simulink model "two_time_domains"  (R2025b)
settings: Solver=ode23tb  StartTime=0.0  StopTime=simlength  MaxStep=tc
undefined symbols (not defined in the file): dead_time_AFE, enable_pwm_phase_corrections, fPWM_AFE, fPWM_INV, ki_align, kp_align, lim_down_align, lim_up_align, omega_base, tc, time_gain_afe_module_1, time_gain_afe_module_2, time_gain_inv_module_1, time_gain_inv_module_2, trgo_th_generator, ts_afe, ts_inv
settings Model: Creator=dbagn  LastModifiedBy=dbagn
settings SolverCC: NumberNewtonIterations=3.0  ZeroCrossControl=DisableAll  AlgebraicLoopSolver=TrustRegion  SolverResetMethod=Robust  AutoInsertRateTranBlk=on
settings DataIOCC: SaveOutput=off  SignalLogging=off  DSMLogging=off  SaveTime=off  ReturnWorkspaceOutputs=off
settings OptimizationCC: ReuseModelBlockBuffer=off
settings DebuggingCC: UnconnectedInputMsg=warning  UnconnectedOutputMsg=warning  UnconnectedLineMsg=warning
settings ModelReferenceCC: UpdateModelReferenceTargets=Force  EnableRefExpFcnMdlSchedulingChecks=on  ParallelModelReferenceMATLABWorkerInit=Copy Base Workspace
settings SFSimCC: CustomCodeUndefinedFunction=ThrowError  DefaultCustomCodeDeterministicFunctions=All
settings RTWCC: GPUComputeCapability=3.5  DLArmComputeVersion=19.05

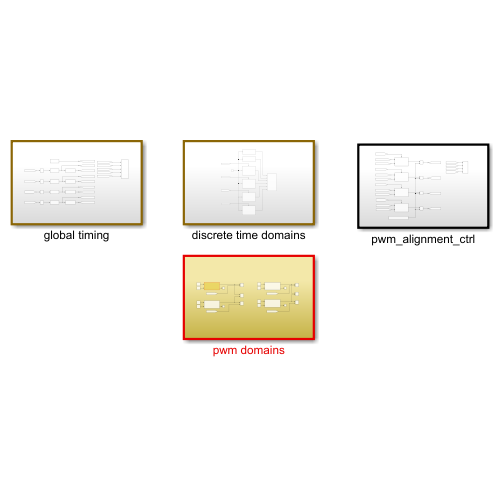
[thumbnail: Simulink's stored preview of the top-level diagram]
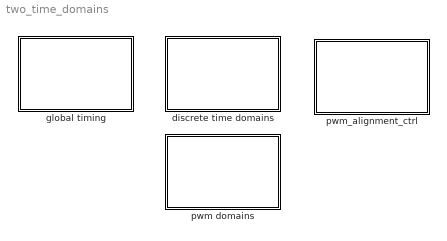
== system two_time_domains ==
  discrete time domains : Subsystem
  global timing : Subsystem
  pwm domains : Subsystem
  pwm_alignment_ctrl : Subsystem

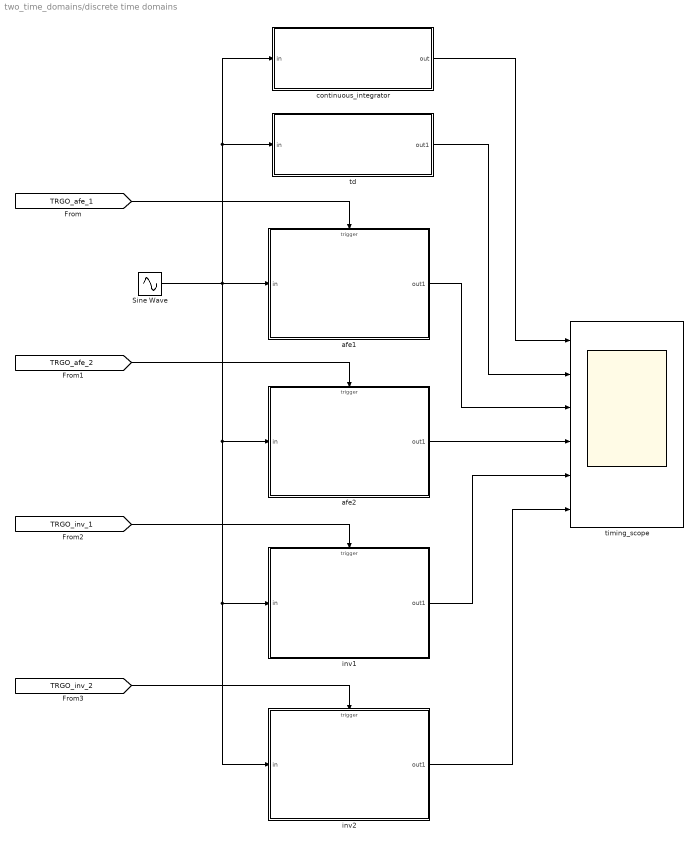
== system two_time_domains/discrete time domains ==
  Sine Wave : Sin  Frequency=omega_base  SampleTime=0
  afe1 : Subsystem
  afe2 : Subsystem
  continuous_integrator : Subsystem
  inv1 : Subsystem
  inv2 : Subsystem
  td : Subsystem
  timing_scope : Scope  NumInputPorts=6
      settings: SampleTime=tc  ActiveDisplayYMinimum=-1.2455953752901299  ActiveDisplayYMaximum=1.2309135739886372
  wires:
  [TRGO_afe_1] -> afe1/Trigger
  [TRGO_afe_2] -> afe2/Trigger
  Sine Wave/1 -> td/1(in), continuous_integrator/1(in), afe1/1(in), inv2/1(in), inv1/1(in), afe2/1(in)
  [TRGO_inv_2] -> inv2/Trigger
  [TRGO_inv_1] -> inv1/Trigger
  afe1/1(out1) -> timing_scope/3
  afe2/1(out1) -> timing_scope/4
  inv1/1(out1) -> timing_scope/5
  inv2/1(out1) -> timing_scope/6
  td/1(out1) -> timing_scope/2
  continuous_integrator/1(out) -> timing_scope/1

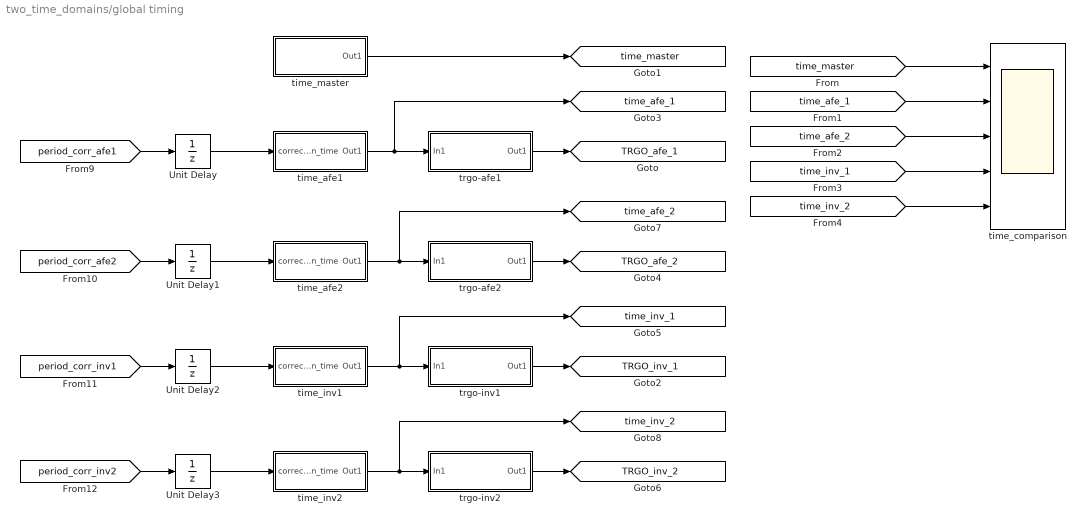
== system two_time_domains/global timing ==
  Unit Delay{,1..3} (4 alike) : UnitDelay  SampleTime=tc  HasFrameUpgradeWarning=on
  time_afe1 : Subsystem  mask{k=time_gain_afe_module_1}
      mask prompts: k "Time Gain"
      mask Display:
      | disp('time-gen');
      | port_label('input', 1, 'crt');
      | port_label('output', 1, 'tout');
  time_afe2 : Subsystem  mask{k=time_gain_afe_module_2}
      mask prompts: k "Time Gain"
      mask Display:
      | disp('time-gen');
      | port_label('input', 1, 'crt');
      | port_label('output', 1, 'tout');
  time_comparison : Scope  NumInputPorts=5
      settings: ActiveDisplayYMinimum=-0.0261093772199036  ActiveDisplayYMaximum=0.23498439497913245  DataLoggingVariableName=ScopeData6
  time_inv1 : Subsystem  mask{k=time_gain_inv_module_1}
      mask prompts: k "Time Gain"
      mask Display:
      | disp('time-gen');
      | port_label('input', 1, 'crt');
      | port_label('output', 1, 'tout');
  time_inv2 : Subsystem  mask{k=time_gain_inv_module_2}
      mask prompts: k "Time Gain"
      mask Display:
      | disp('time-gen');
      | port_label('input', 1, 'crt');
      | port_label('output', 1, 'tout');
  time_master : Subsystem  mask{k=1}
      mask prompts: k "Time Gain"
      mask Display:
      | disp('master');
      | port_label('output', 1, 'time');
  trgo-afe1 : Subsystem  mask{samplig_time=ts_afe}
      mask prompts: samplig_time "Sampling Time"
      mask Display: disp('TRGO Generator');
  trgo-afe2 : Subsystem  mask{samplig_time=ts_afe}
      mask prompts: samplig_time "Sampling Time"
      mask Display: disp('TRGO Generator');
  trgo-inv1 : Subsystem  mask{samplig_time=ts_inv}
      mask prompts: samplig_time "Sampling Time"
      mask Display: disp('TRGO Generator');
  trgo-inv2 : Subsystem  mask{samplig_time=ts_inv}
      mask prompts: samplig_time "Sampling Time"
      mask Display: disp('TRGO Generator');
  tag scope: TRGO_afe_1=global, TRGO_afe_2=global, TRGO_inv_1=global, TRGO_inv_2=global, time_afe_1=global, time_afe_2=global, time_inv_1=global, time_inv_2=global, time_master=global
  wires:
  time_afe1/1(Out1) -> [time_afe_1], trgo-afe1/1(In1)
  trgo-afe1/1(Out1) -> [TRGO_afe_1]
  trgo-afe2/1(Out1) -> [TRGO_afe_2]
  time_afe2/1(Out1) -> trgo-afe2/1(In1), [time_afe_2]
  time_master/1(Out1) -> [time_master]
  time_inv2/1(Out1) -> [time_inv_2], trgo-inv2/1(In1)
  trgo-inv2/1(Out1) -> [TRGO_inv_2]
  trgo-inv1/1(Out1) -> [TRGO_inv_1]
  time_inv1/1(Out1) -> trgo-inv1/1(In1), [time_inv_1]
  Unit Delay/1 -> time_afe1/1(correction_time)
  Unit Delay1/1 -> time_afe2/1(correction_time)
  Unit Delay2/1 -> time_inv1/1(correction_time)
  Unit Delay3/1 -> time_inv2/1(correction_time)
  [time_master] -> time_comparison/1
  [time_afe_1] -> time_comparison/2
  [time_afe_2] -> time_comparison/3
  [time_inv_1] -> time_comparison/4
  [time_inv_2] -> time_comparison/5
  [period_corr_inv2] -> Unit Delay3/1
  [period_corr_inv1] -> Unit Delay2/1
  [period_corr_afe2] -> Unit Delay1/1
  [period_corr_afe1] -> Unit Delay/1

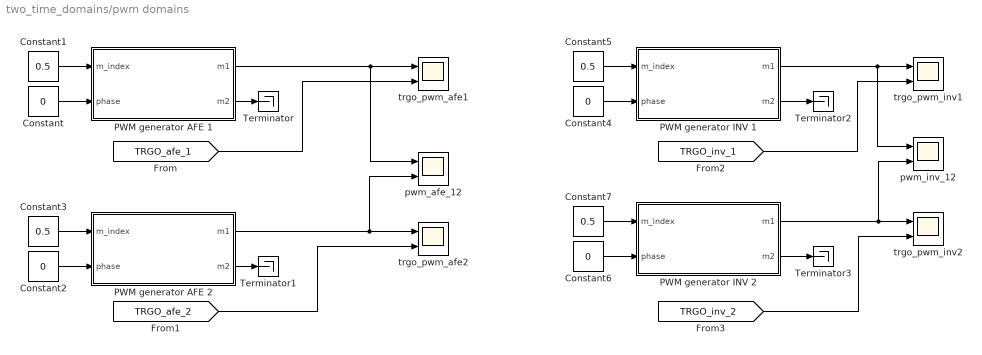
== system two_time_domains/pwm domains ==
  Constant{,2,4,6} (4 alike) : Constant  Value=0
  Constant{1,3,5,7} (4 alike) : Constant  Value=0.5
  PWM generator AFE 1 : Subsystem  mask{f=fPWM_AFE, m_up=0.98, m_low=0.02, dead_time=dead_time_AFE, pos_cmd_gate=1, neg_cmd_gate=0, polarity=1}
      mask prompts: f "Frequency (Hz)"; m_up "Max Input Modulation Value"; m_low "Min Input Modulation Value"; dead_time "Dead Time (s)"; pos_cmd_gate "Positive Gate Voltage (V)"; neg_cmd_gate "Negative Gate Voltage (V)"; polarity "Polarity (pu)"
  PWM generator AFE 2 : Subsystem  mask{f=fPWM_AFE, m_up=0.98, m_low=0.02, dead_time=dead_time_AFE, pos_cmd_gate=1, neg_cmd_gate=0, polarity=1}
      mask prompts: f "Frequency (Hz)"; m_up "Max Input Modulation Value"; m_low "Min Input Modulation Value"; dead_time "Dead Time (s)"; pos_cmd_gate "Positive Gate Voltage (V)"; neg_cmd_gate "Negative Gate Voltage (V)"; polarity "Polarity (pu)"
  PWM generator INV 1 : Subsystem  mask{f=fPWM_INV, m_up=0.98, m_low=0.02, dead_time=dead_time_AFE, pos_cmd_gate=1, neg_cmd_gate=0, polarity=1}
      mask prompts: f "Frequency (Hz)"; m_up "Max Input Modulation Value"; m_low "Min Input Modulation Value"; dead_time "Dead Time (s)"; pos_cmd_gate "Positive Gate Voltage (V)"; neg_cmd_gate "Negative Gate Voltage (V)"; polarity "Polarity (pu)"
  PWM generator INV 2 : Subsystem  mask{f=fPWM_INV, m_up=0.98, m_low=0.02, dead_time=dead_time_AFE, pos_cmd_gate=1, neg_cmd_gate=0, polarity=1}
      mask prompts: f "Frequency (Hz)"; m_up "Max Input Modulation Value"; m_low "Min Input Modulation Value"; dead_time "Dead Time (s)"; pos_cmd_gate "Positive Gate Voltage (V)"; neg_cmd_gate "Negative Gate Voltage (V)"; polarity "Polarity (pu)"
  Terminator{,1..3} (4 alike) : Terminator
  pwm_afe_12 : Scope  NumInputPorts=2
      settings: ActiveDisplayYMinimum=-0.12499999999999997  ActiveDisplayYMaximum=1.125  DataLoggingVariableName=ScopeData5
  pwm_inv_12 : Scope  NumInputPorts=2
      settings: ActiveDisplayYMinimum=-0.12499999999999997  ActiveDisplayYMaximum=1.125  DataLoggingVariableName=ScopeData8
  trgo_pwm_afe1 : Scope  NumInputPorts=2
      settings: ActiveDisplayYMinimum=-0.12499999999999997  ActiveDisplayYMaximum=1.125
  trgo_pwm_afe2 : Scope  NumInputPorts=2
      settings: ActiveDisplayYMinimum=-0.12499999999999997  ActiveDisplayYMaximum=1.125  DataLoggingVariableName=ScopeData2
  trgo_pwm_inv1 : Scope  NumInputPorts=2
      settings: ActiveDisplayYMinimum=-0.12499999999999997  ActiveDisplayYMaximum=1.125  DataLoggingVariableName=ScopeData3
  trgo_pwm_inv2 : Scope  NumInputPorts=2
      settings: ActiveDisplayYMinimum=-0.12499999999999997  ActiveDisplayYMaximum=1.125  DataLoggingVariableName=ScopeData4
  wires:
  Constant/1 -> PWM generator AFE 1/2(phase)
  Constant1/1 -> PWM generator AFE 1/1(m_index)
  Constant3/1 -> PWM generator AFE 2/1(m_index)
  Constant2/1 -> PWM generator AFE 2/2(phase)
  Constant7/1 -> PWM generator INV 2/1(m_index)
  Constant5/1 -> PWM generator INV 1/1(m_index)
  Constant4/1 -> PWM generator INV 1/2(phase)
  Constant6/1 -> PWM generator INV 2/2(phase)
  PWM generator AFE 1/1(m1) -> pwm_afe_12/1, trgo_pwm_afe1/1
  [TRGO_afe_1] -> trgo_pwm_afe1/2
  PWM generator AFE 2/1(m1) -> pwm_afe_12/2, trgo_pwm_afe2/1
  [TRGO_afe_2] -> trgo_pwm_afe2/2
  [TRGO_inv_1] -> trgo_pwm_inv1/2
  PWM generator INV 1/1(m1) -> pwm_inv_12/1, trgo_pwm_inv1/1
  PWM generator INV 2/1(m1) -> pwm_inv_12/2, trgo_pwm_inv2/1
  [TRGO_inv_2] -> trgo_pwm_inv2/2
  PWM generator AFE 1/2(m2) -> Terminator/1
  PWM generator AFE 2/2(m2) -> Terminator1/1
  PWM generator INV 1/2(m2) -> Terminator2/1
  PWM generator INV 2/2(m2) -> Terminator3/1

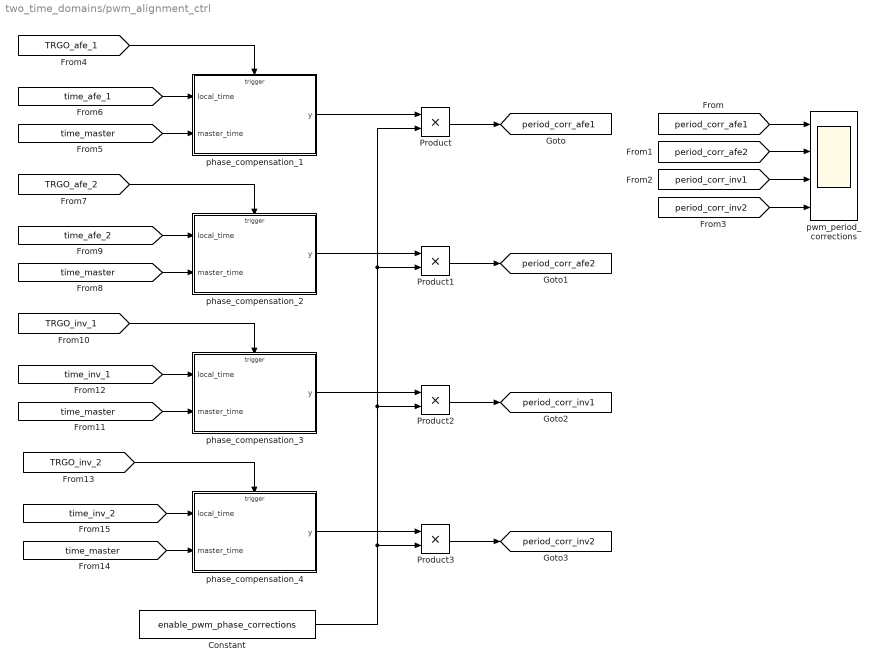
== system two_time_domains/pwm_alignment_ctrl ==
  Constant : Constant  Value=enable_pwm_phase_corrections
  Product{,1..3} (4 alike) : Product
  phase_compensation_1 : Subsystem
  phase_compensation_2 : Subsystem
  phase_compensation_3 : Subsystem
  phase_compensation_4 : Subsystem
  pwm_period_corrections : Scope  NumInputPorts=4
      settings: ActiveDisplayYMinimum=-0.12053571417135155  ActiveDisplayYMaximum=0.013392857130150168  DataLoggingVariableName=ScopeData7
  tag scope: period_corr_afe1=global, period_corr_afe2=global, period_corr_inv1=global, period_corr_inv2=global
  wires:
  Constant/1 -> Product1/2, Product/2, Product2/2, Product3/2
  Product/1 -> [period_corr_afe1]
  Product1/1 -> [period_corr_afe2]
  Product2/1 -> [period_corr_inv1]
  Product3/1 -> [period_corr_inv2]
  [period_corr_afe1] -> pwm_period_corrections/1
  [period_corr_afe2] -> pwm_period_corrections/2
  [period_corr_inv1] -> pwm_period_corrections/3
  [period_corr_inv2] -> pwm_period_corrections/4
  phase_compensation_1/1(y) -> Product/1
  [time_afe_1] -> phase_compensation_1/1(local_time)
  [time_master] -> phase_compensation_1/2(master_time)
  [time_master] -> phase_compensation_2/2(master_time)
  [time_afe_2] -> phase_compensation_2/1(local_time)
  phase_compensation_2/1(y) -> Product1/1
  [time_inv_1] -> phase_compensation_3/1(local_time)
  [time_master] -> phase_compensation_3/2(master_time)
  phase_compensation_3/1(y) -> Product2/1
  [time_master] -> phase_compensation_4/2(master_time)
  [time_inv_2] -> phase_compensation_4/1(local_time)
  phase_compensation_4/1(y) -> Product3/1
  [TRGO_afe_1] -> phase_compensation_1/Trigger
  [TRGO_inv_2] -> phase_compensation_4/Trigger
  [TRGO_inv_1] -> phase_compensation_3/Trigger
  [TRGO_afe_2] -> phase_compensation_2/Trigger

== system two_time_domains/discrete time domains/afe1 ==
  in : Inport
  Trigger : TriggerPort  VariantControl=(inherit)  PortDimensions=1
  LPF1_1 : Subsystem  mask{ts=ts_afe, omega=omega_base}
      mask Display:
      | disp('LPF1');
      | port_label('input', 1, 'u');
      | port_label('output', 1, 'y');
  out1 : Outport
  wires:
  in/1 -> LPF1_1/1(u)
  LPF1_1/1(y) -> out1/1

== system two_time_domains/discrete time domains/afe2 ==
  in : Inport
  Trigger : TriggerPort  VariantControl=(inherit)  PortDimensions=1
  LPF1_1 : Subsystem  mask{ts=ts_afe, omega=omega_base}
      mask Display:
      | disp('LPF1');
      | port_label('input', 1, 'u');
      | port_label('output', 1, 'y');
  out1 : Outport
  wires:
  LPF1_1/1(y) -> out1/1
  in/1 -> LPF1_1/1(u)

== system two_time_domains/discrete time domains/continuous_integrator ==
  in : Inport
  Transfer Fcn : TransferFcn  Denominator=[1/omega_base 1]
  out : Outport
  wires:
  in/1 -> Transfer Fcn/1
  Transfer Fcn/1 -> out/1

== system two_time_domains/discrete time domains/inv1 ==
  in : Inport
  Trigger : TriggerPort  VariantControl=(inherit)  PortDimensions=1
  LPF1_1 : Subsystem  mask{ts=ts_inv, omega=omega_base}
      mask Display:
      | disp('LPF1');
      | port_label('input', 1, 'u');
      | port_label('output', 1, 'y');
  out1 : Outport
  wires:
  in/1 -> LPF1_1/1(u)
  LPF1_1/1(y) -> out1/1

== system two_time_domains/discrete time domains/inv2 ==
  in : Inport
  Trigger : TriggerPort  VariantControl=(inherit)  PortDimensions=1
  LPF1_1 : Subsystem  mask{ts=ts_inv, omega=omega_base}
      mask Display:
      | disp('LPF1');
      | port_label('input', 1, 'u');
      | port_label('output', 1, 'y');
  out1 : Outport
  wires:
  LPF1_1/1(y) -> out1/1
  in/1 -> LPF1_1/1(u)

== system two_time_domains/discrete time domains/td ==
  in : Inport
  LPF1_1 : Subsystem  mask{ts=tc, omega=omega_base}
      mask Display:
      | disp('LPF1');
      | port_label('input', 1, 'u');
      | port_label('output', 1, 'y');
  out1 : Outport
  wires:
  LPF1_1/1(y) -> out1/1
  in/1 -> LPF1_1/1(u)

== system two_time_domains/global timing/time_afe1 ==
  correction_time : Inport
  Constant : Constant
  Gain : Gain  Gain=k
  Product : Product
  Sum : Sum  Inputs=|++
  time_1 : Clock
  Out1 : Outport
  wires:
  time_1/1 -> Gain/1
  Gain/1 -> Product/1
  Product/1 -> Out1/1
  correction_time/1 -> Sum/1
  Sum/1 -> Product/2
  Constant/1 -> Sum/2

== system two_time_domains/global timing/time_afe2 ==
  correction_time : Inport
  Constant : Constant
  Gain : Gain  Gain=k
  Product : Product
  Sum : Sum  Inputs=|++
  time_1 : Clock
  Out1 : Outport
  wires:
  time_1/1 -> Gain/1
  Gain/1 -> Product/1
  Product/1 -> Out1/1
  correction_time/1 -> Sum/1
  Constant/1 -> Sum/2
  Sum/1 -> Product/2

== system two_time_domains/global timing/time_inv1 ==
  correction_time : Inport
  Constant : Constant
  Gain : Gain  Gain=k
  Product : Product
  Sum : Sum  Inputs=|++
  time_1 : Clock
  Out1 : Outport
  wires:
  time_1/1 -> Gain/1
  Gain/1 -> Product/1
  Product/1 -> Out1/1
  correction_time/1 -> Sum/1
  Constant/1 -> Sum/2
  Sum/1 -> Product/2

== system two_time_domains/global timing/time_inv2 ==
  correction_time : Inport
  Constant : Constant
  Gain : Gain  Gain=k
  Product : Product
  Sum : Sum  Inputs=|++
  time_1 : Clock
  Out1 : Outport
  wires:
  time_1/1 -> Gain/1
  Gain/1 -> Product/1
  Product/1 -> Out1/1
  correction_time/1 -> Sum/1
  Constant/1 -> Sum/2
  Sum/1 -> Product/2

== system two_time_domains/global timing/time_master ==
  Gain : Gain  Gain=k
  time_1 : Clock
  Out1 : Outport
  wires:
  Gain/1 -> Out1/1
  time_1/1 -> Gain/1

== system two_time_domains/global timing/trgo-afe1 ==
  In1 : Inport
  Constant1 : Constant  Value=samplig_time
  Gain2 : Gain  Gain=1/samplig_time
  Mod1 : Math  Operator=mod
  schmitt : Subsystem
  Out1 : Outport
  wires:
  Constant1/1 -> Mod1/2
  In1/1 -> Mod1/1
  Mod1/1 -> Gain2/1
  schmitt/1(Out1) -> Out1/1
  Gain2/1 -> schmitt/1(In1)

== system two_time_domains/global timing/trgo-afe2 ==
  In1 : Inport
  Constant1 : Constant  Value=samplig_time
  Gain2 : Gain  Gain=1/samplig_time
  Mod1 : Math  Operator=mod
  schmitt : Subsystem
  Out1 : Outport
  wires:
  Gain2/1 -> schmitt/1(In1)
  schmitt/1(Out1) -> Out1/1
  Mod1/1 -> Gain2/1
  In1/1 -> Mod1/1
  Constant1/1 -> Mod1/2

== system two_time_domains/global timing/trgo-inv1 ==
  In1 : Inport
  Constant1 : Constant  Value=samplig_time
  Gain2 : Gain  Gain=1/samplig_time
  Mod1 : Math  Operator=mod
  schmitt : Subsystem
  Out1 : Outport
  wires:
  Gain2/1 -> schmitt/1(In1)
  schmitt/1(Out1) -> Out1/1
  Mod1/1 -> Gain2/1
  In1/1 -> Mod1/1
  Constant1/1 -> Mod1/2

== system two_time_domains/global timing/trgo-inv2 ==
  In1 : Inport
  Constant1 : Constant  Value=samplig_time
  Gain2 : Gain  Gain=1/samplig_time
  Mod1 : Math  Operator=mod
  schmitt : Subsystem
  Out1 : Outport
  wires:
  Constant1/1 -> Mod1/2
  In1/1 -> Mod1/1
  Mod1/1 -> Gain2/1
  schmitt/1(Out1) -> Out1/1
  Gain2/1 -> schmitt/1(In1)

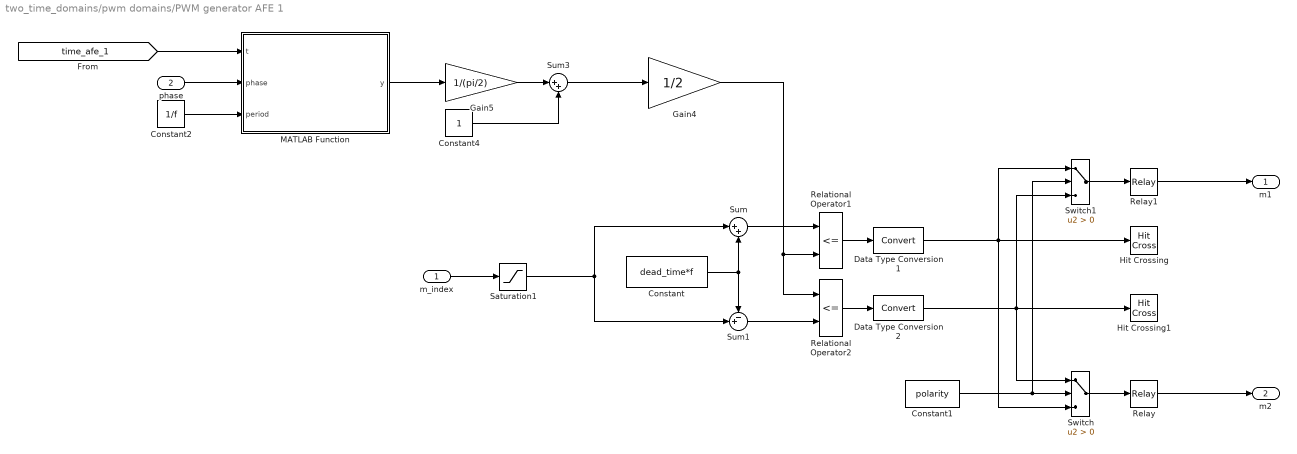
== system two_time_domains/pwm domains/PWM generator AFE 1 ==
  m_index : Inport
  phase : Inport  Port=2
  Constant : Constant  Value=dead_time*f
  Constant1 : Constant  Value=polarity
  Constant2 : Constant  Value=1/f
  Constant4 : Constant
  Data Type Conversion1 : DataTypeConversion
  Data Type Conversion2 : DataTypeConversion
  Gain4 : Gain  Gain=1/2
  Gain5 : Gain  Gain=1/(pi/2)
  Hit Crossing : HitCross  ShowOutputPort=off
  Hit Crossing1 : HitCross  ShowOutputPort=off
  MATLAB Function : MATLAB Function  TreatAsAtomicUnit=on
  Relational Operator1 : RelationalOperator  Operator=<=  InputSameDT=off
  Relational Operator2 : RelationalOperator  Operator=<=  InputSameDT=off
  Relay : Relay  OnOutputValue=pos_cmd_gate  OffOutputValue=neg_cmd_gate
  Relay1 : Relay  OnOutputValue=pos_cmd_gate  OffOutputValue=neg_cmd_gate
  Saturation1 : Saturate  UpperLimit=m_up  LowerLimit=m_low
  Sum : Sum  Inputs=|++  SaturateOnIntegerOverflow=on
  Sum1 : Sum  Inputs=-+|  SaturateOnIntegerOverflow=on
  Sum3 : Sum  Inputs=|++
  Switch : Switch  Criteria=u2 > Threshold  SaturateOnIntegerOverflow=off  InputSameDT=off
  Switch1 : Switch  Criteria=u2 > Threshold  SaturateOnIntegerOverflow=off  InputSameDT=off
  m1 : Outport
  m2 : Outport  Port=2
  wires:
  Relational Operator1/1 -> Data Type Conversion1/1
  m_index/1 -> Saturation1/1
  Relational Operator2/1 -> Data Type Conversion2/1
  Data Type Conversion2/1 -> Switch/1, Switch1/3, Hit Crossing1/1
  Constant/1 -> Sum/2, Sum1/1
  Saturation1/1 -> Sum/1, Sum1/2
  Sum/1 -> Relational Operator1/1
  Sum1/1 -> Relational Operator2/2
  Gain4/1 -> Relational Operator2/1, Relational Operator1/2
  Data Type Conversion1/1 -> Hit Crossing/1, Switch/3, Switch1/1
  Switch/1 -> Relay/1
  Constant2/1 -> MATLAB Function/3(period)
  phase/1 -> MATLAB Function/2(phase)
  MATLAB Function/1(y) -> Gain5/1
  Gain5/1 -> Sum3/1
  Sum3/1 -> Gain4/1
  Constant4/1 -> Sum3/2
  Relay/1 -> m2/1
  Constant1/1 -> Switch1/2, Switch/2
  Switch1/1 -> Relay1/1
  Relay1/1 -> m1/1
  [time_afe_1] -> MATLAB Function/1(t)

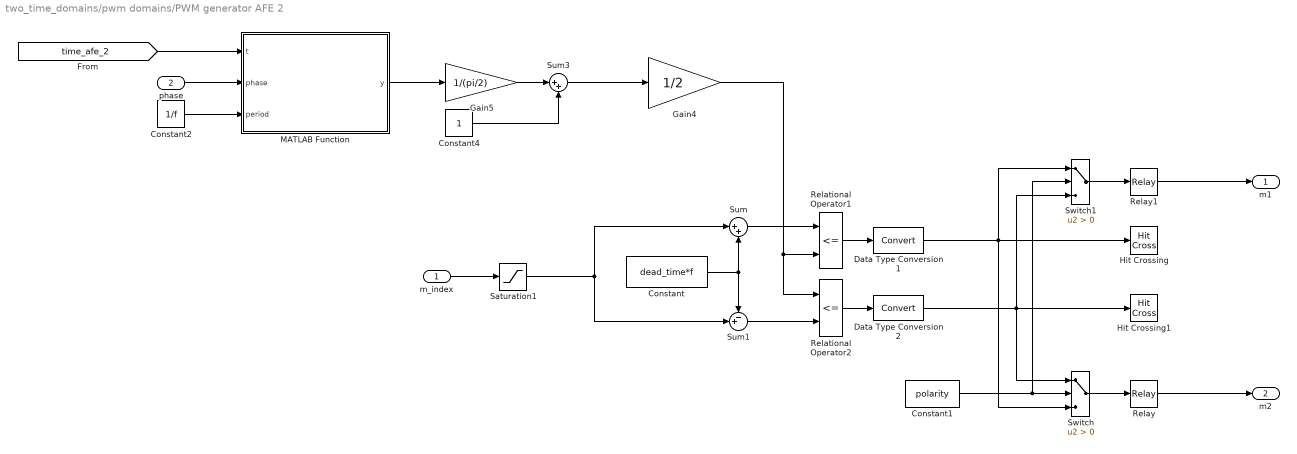
== system two_time_domains/pwm domains/PWM generator AFE 2 ==
  m_index : Inport
  phase : Inport  Port=2
  Constant : Constant  Value=dead_time*f
  Constant1 : Constant  Value=polarity
  Constant2 : Constant  Value=1/f
  Constant4 : Constant
  Data Type Conversion1 : DataTypeConversion
  Data Type Conversion2 : DataTypeConversion
  Gain4 : Gain  Gain=1/2
  Gain5 : Gain  Gain=1/(pi/2)
  Hit Crossing : HitCross  ShowOutputPort=off
  Hit Crossing1 : HitCross  ShowOutputPort=off
  MATLAB Function : MATLAB Function  TreatAsAtomicUnit=on
  Relational Operator1 : RelationalOperator  Operator=<=  InputSameDT=off
  Relational Operator2 : RelationalOperator  Operator=<=  InputSameDT=off
  Relay : Relay  OnOutputValue=pos_cmd_gate  OffOutputValue=neg_cmd_gate
  Relay1 : Relay  OnOutputValue=pos_cmd_gate  OffOutputValue=neg_cmd_gate
  Saturation1 : Saturate  UpperLimit=m_up  LowerLimit=m_low
  Sum : Sum  Inputs=|++  SaturateOnIntegerOverflow=on
  Sum1 : Sum  Inputs=-+|  SaturateOnIntegerOverflow=on
  Sum3 : Sum  Inputs=|++
  Switch : Switch  Criteria=u2 > Threshold  SaturateOnIntegerOverflow=off  InputSameDT=off
  Switch1 : Switch  Criteria=u2 > Threshold  SaturateOnIntegerOverflow=off  InputSameDT=off
  m1 : Outport
  m2 : Outport  Port=2
  wires:
  [time_afe_2] -> MATLAB Function/1(t)
  Relay1/1 -> m1/1
  Switch1/1 -> Relay1/1
  Constant1/1 -> Switch/2, Switch1/2
  Relay/1 -> m2/1
  Constant4/1 -> Sum3/2
  Sum3/1 -> Gain4/1
  Gain5/1 -> Sum3/1
  MATLAB Function/1(y) -> Gain5/1
  phase/1 -> MATLAB Function/2(phase)
  Constant2/1 -> MATLAB Function/3(period)
  Switch/1 -> Relay/1
  Data Type Conversion1/1 -> Switch1/1, Switch/3, Hit Crossing/1
  Gain4/1 -> Relational Operator1/2, Relational Operator2/1
  Sum1/1 -> Relational Operator2/2
  Sum/1 -> Relational Operator1/1
  Saturation1/1 -> Sum1/2, Sum/1
  Constant/1 -> Sum1/1, Sum/2
  Data Type Conversion2/1 -> Hit Crossing1/1, Switch1/3, Switch/1
  Relational Operator2/1 -> Data Type Conversion2/1
  m_index/1 -> Saturation1/1
  Relational Operator1/1 -> Data Type Conversion1/1

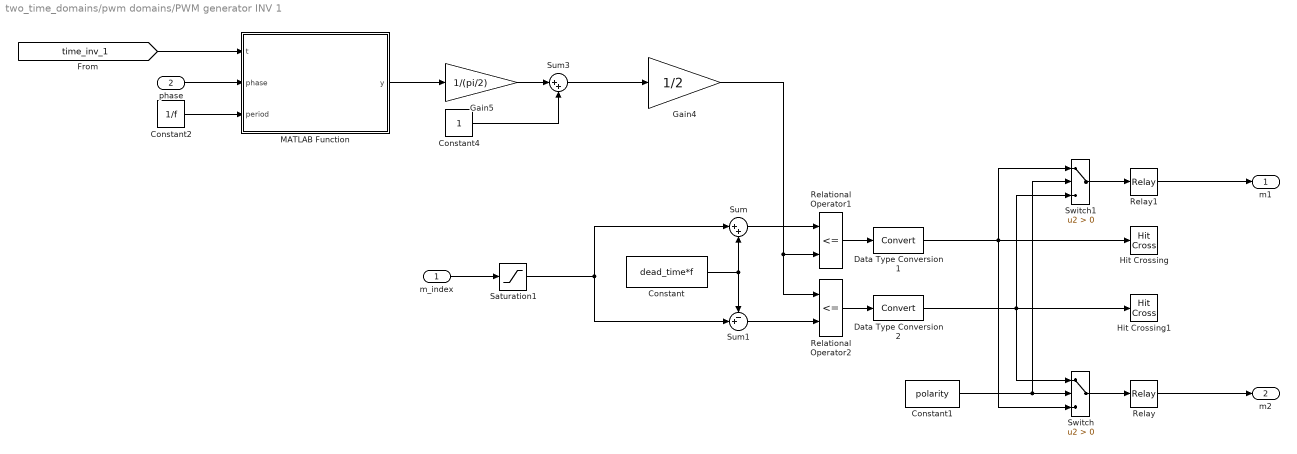
== system two_time_domains/pwm domains/PWM generator INV 1 ==
  m_index : Inport
  phase : Inport  Port=2
  Constant : Constant  Value=dead_time*f
  Constant1 : Constant  Value=polarity
  Constant2 : Constant  Value=1/f
  Constant4 : Constant
  Data Type Conversion1 : DataTypeConversion
  Data Type Conversion2 : DataTypeConversion
  Gain4 : Gain  Gain=1/2
  Gain5 : Gain  Gain=1/(pi/2)
  Hit Crossing : HitCross  ShowOutputPort=off
  Hit Crossing1 : HitCross  ShowOutputPort=off
  MATLAB Function : MATLAB Function  TreatAsAtomicUnit=on
  Relational Operator1 : RelationalOperator  Operator=<=  InputSameDT=off
  Relational Operator2 : RelationalOperator  Operator=<=  InputSameDT=off
  Relay : Relay  OnOutputValue=pos_cmd_gate  OffOutputValue=neg_cmd_gate
  Relay1 : Relay  OnOutputValue=pos_cmd_gate  OffOutputValue=neg_cmd_gate
  Saturation1 : Saturate  UpperLimit=m_up  LowerLimit=m_low
  Sum : Sum  Inputs=|++  SaturateOnIntegerOverflow=on
  Sum1 : Sum  Inputs=-+|  SaturateOnIntegerOverflow=on
  Sum3 : Sum  Inputs=|++
  Switch : Switch  Criteria=u2 > Threshold  SaturateOnIntegerOverflow=off  InputSameDT=off
  Switch1 : Switch  Criteria=u2 > Threshold  SaturateOnIntegerOverflow=off  InputSameDT=off
  m1 : Outport
  m2 : Outport  Port=2
  wires:
  [time_inv_1] -> MATLAB Function/1(t)
  Relay1/1 -> m1/1
  Switch1/1 -> Relay1/1
  Constant1/1 -> Switch/2, Switch1/2
  Relay/1 -> m2/1
  Constant4/1 -> Sum3/2
  Sum3/1 -> Gain4/1
  Gain5/1 -> Sum3/1
  MATLAB Function/1(y) -> Gain5/1
  phase/1 -> MATLAB Function/2(phase)
  Constant2/1 -> MATLAB Function/3(period)
  Switch/1 -> Relay/1
  Data Type Conversion1/1 -> Switch1/1, Switch/3, Hit Crossing/1
  Gain4/1 -> Relational Operator1/2, Relational Operator2/1
  Sum1/1 -> Relational Operator2/2
  Sum/1 -> Relational Operator1/1
  Saturation1/1 -> Sum1/2, Sum/1
  Constant/1 -> Sum1/1, Sum/2
  Data Type Conversion2/1 -> Hit Crossing1/1, Switch1/3, Switch/1
  Relational Operator2/1 -> Data Type Conversion2/1
  m_index/1 -> Saturation1/1
  Relational Operator1/1 -> Data Type Conversion1/1

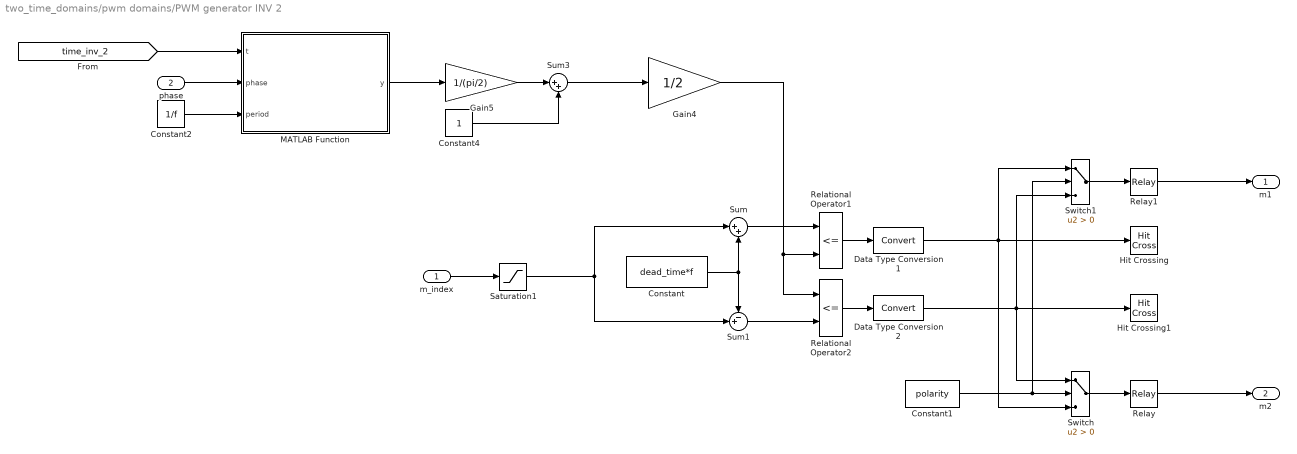
== system two_time_domains/pwm domains/PWM generator INV 2 ==
  m_index : Inport
  phase : Inport  Port=2
  Constant : Constant  Value=dead_time*f
  Constant1 : Constant  Value=polarity
  Constant2 : Constant  Value=1/f
  Constant4 : Constant
  Data Type Conversion1 : DataTypeConversion
  Data Type Conversion2 : DataTypeConversion
  Gain4 : Gain  Gain=1/2
  Gain5 : Gain  Gain=1/(pi/2)
  Hit Crossing : HitCross  ShowOutputPort=off
  Hit Crossing1 : HitCross  ShowOutputPort=off
  MATLAB Function : MATLAB Function  TreatAsAtomicUnit=on
  Relational Operator1 : RelationalOperator  Operator=<=  InputSameDT=off
  Relational Operator2 : RelationalOperator  Operator=<=  InputSameDT=off
  Relay : Relay  OnOutputValue=pos_cmd_gate  OffOutputValue=neg_cmd_gate
  Relay1 : Relay  OnOutputValue=pos_cmd_gate  OffOutputValue=neg_cmd_gate
  Saturation1 : Saturate  UpperLimit=m_up  LowerLimit=m_low
  Sum : Sum  Inputs=|++  SaturateOnIntegerOverflow=on
  Sum1 : Sum  Inputs=-+|  SaturateOnIntegerOverflow=on
  Sum3 : Sum  Inputs=|++
  Switch : Switch  Criteria=u2 > Threshold  SaturateOnIntegerOverflow=off  InputSameDT=off
  Switch1 : Switch  Criteria=u2 > Threshold  SaturateOnIntegerOverflow=off  InputSameDT=off
  m1 : Outport
  m2 : Outport  Port=2
  wires:
  Relational Operator1/1 -> Data Type Conversion1/1
  m_index/1 -> Saturation1/1
  Relational Operator2/1 -> Data Type Conversion2/1
  Data Type Conversion2/1 -> Switch/1, Switch1/3, Hit Crossing1/1
  Constant/1 -> Sum/2, Sum1/1
  Saturation1/1 -> Sum/1, Sum1/2
  Sum/1 -> Relational Operator1/1
  Sum1/1 -> Relational Operator2/2
  Gain4/1 -> Relational Operator2/1, Relational Operator1/2
  Data Type Conversion1/1 -> Hit Crossing/1, Switch/3, Switch1/1
  Switch/1 -> Relay/1
  Constant2/1 -> MATLAB Function/3(period)
  phase/1 -> MATLAB Function/2(phase)
  MATLAB Function/1(y) -> Gain5/1
  Gain5/1 -> Sum3/1
  Sum3/1 -> Gain4/1
  Constant4/1 -> Sum3/2
  Relay/1 -> m2/1
  Constant1/1 -> Switch1/2, Switch/2
  Switch1/1 -> Relay1/1
  Relay1/1 -> m1/1
  [time_inv_2] -> MATLAB Function/1(t)

== system two_time_domains/pwm_alignment_ctrl/phase_compensation_1 ==
  local_time : Inport
  master_time : Inport  Port=2
  Trigger : TriggerPort  VariantControl=(inherit)  PortDimensions=1
  alignment_eval_afe1 : Subsystem
  y : Outport
  wires:
  local_time/1 -> alignment_eval_afe1/1(local_time)
  master_time/1 -> alignment_eval_afe1/2(master_time)
  alignment_eval_afe1/1(dp) -> y/1

== system two_time_domains/pwm_alignment_ctrl/phase_compensation_2 ==
  local_time : Inport
  master_time : Inport  Port=2
  Trigger : TriggerPort  VariantControl=(inherit)  PortDimensions=1
  alignment_eval_afe1 : Subsystem
  y : Outport
  wires:
  alignment_eval_afe1/1(dp) -> y/1
  master_time/1 -> alignment_eval_afe1/2(master_time)
  local_time/1 -> alignment_eval_afe1/1(local_time)

== system two_time_domains/pwm_alignment_ctrl/phase_compensation_3 ==
  local_time : Inport
  master_time : Inport  Port=2
  Trigger : TriggerPort  VariantControl=(inherit)  PortDimensions=1
  alignment_eval_afe1 : Subsystem
  y : Outport
  wires:
  local_time/1 -> alignment_eval_afe1/1(local_time)
  master_time/1 -> alignment_eval_afe1/2(master_time)
  alignment_eval_afe1/1(dp) -> y/1

== system two_time_domains/pwm_alignment_ctrl/phase_compensation_4 ==
  local_time : Inport
  master_time : Inport  Port=2
  Trigger : TriggerPort  VariantControl=(inherit)  PortDimensions=1
  alignment_eval_afe1 : Subsystem
  y : Outport
  wires:
  alignment_eval_afe1/1(dp) -> y/1
  master_time/1 -> alignment_eval_afe1/2(master_time)
  local_time/1 -> alignment_eval_afe1/1(local_time)

== system two_time_domains/discrete time domains/afe1/LPF1_1 ==
  u : Inport
  Gain : Gain  Gain=1-exp(-omega*ts)
  Gain1 : Gain  Gain=exp(-omega*ts)
  Sum : Sum  Inputs=|++
  Unit Delay : UnitDelay  SampleTime=-1  HasFrameUpgradeWarning=on
  y : Outport
  wires:
  Gain1/1 -> Sum/2
  Unit Delay/1 -> y/1, Gain1/1
  Gain/1 -> Sum/1
  Sum/1 -> Unit Delay/1
  u/1 -> Gain/1

== system two_time_domains/discrete time domains/afe2/LPF1_1 ==
  u : Inport
  Gain : Gain  Gain=1-exp(-omega*ts)
  Gain1 : Gain  Gain=exp(-omega*ts)
  Sum : Sum  Inputs=|++
  Unit Delay : UnitDelay  SampleTime=-1  HasFrameUpgradeWarning=on
  y : Outport
  wires:
  u/1 -> Gain/1
  Sum/1 -> Unit Delay/1
  Gain/1 -> Sum/1
  Unit Delay/1 -> Gain1/1, y/1
  Gain1/1 -> Sum/2

== system two_time_domains/discrete time domains/inv1/LPF1_1 ==
  u : Inport
  Gain : Gain  Gain=1-exp(-omega*ts)
  Gain1 : Gain  Gain=exp(-omega*ts)
  Sum : Sum  Inputs=|++
  Unit Delay : UnitDelay  SampleTime=-1  HasFrameUpgradeWarning=on
  y : Outport
  wires:
  Gain1/1 -> Sum/2
  Unit Delay/1 -> y/1, Gain1/1
  Gain/1 -> Sum/1
  Sum/1 -> Unit Delay/1
  u/1 -> Gain/1

== system two_time_domains/discrete time domains/inv2/LPF1_1 ==
  u : Inport
  Gain : Gain  Gain=1-exp(-omega*ts)
  Gain1 : Gain  Gain=exp(-omega*ts)
  Sum : Sum  Inputs=|++
  Unit Delay : UnitDelay  SampleTime=-1  HasFrameUpgradeWarning=on
  y : Outport
  wires:
  u/1 -> Gain/1
  Sum/1 -> Unit Delay/1
  Gain/1 -> Sum/1
  Unit Delay/1 -> Gain1/1, y/1
  Gain1/1 -> Sum/2

== system two_time_domains/discrete time domains/td/LPF1_1 ==
  u : Inport
  Gain : Gain  Gain=1-exp(-omega*ts)
  Gain1 : Gain  Gain=exp(-omega*ts)
  Sum : Sum  Inputs=|++
  Unit Delay : UnitDelay  SampleTime=-1  HasFrameUpgradeWarning=on
  y : Outport
  wires:
  u/1 -> Gain/1
  Sum/1 -> Unit Delay/1
  Gain/1 -> Sum/1
  Unit Delay/1 -> Gain1/1, y/1
  Gain1/1 -> Sum/2

== system two_time_domains/global timing/trgo-afe1/schmitt ==
  In1 : Inport
  Constant2 : Constant
  Constant3 : Constant  Value=0
  Switch : Switch  Threshold=trgo_th_generator  SaturateOnIntegerOverflow=off  InputSameDT=off
  Out1 : Outport
  wires:
  Constant2/1 -> Switch/3
  Constant3/1 -> Switch/1
  In1/1 -> Switch/2
  Switch/1 -> Out1/1

== system two_time_domains/global timing/trgo-afe2/schmitt ==
  In1 : Inport
  Constant2 : Constant
  Constant3 : Constant  Value=0
  Switch : Switch  Threshold=trgo_th_generator  SaturateOnIntegerOverflow=off  InputSameDT=off
  Out1 : Outport
  wires:
  Switch/1 -> Out1/1
  In1/1 -> Switch/2
  Constant3/1 -> Switch/1
  Constant2/1 -> Switch/3

== system two_time_domains/global timing/trgo-inv1/schmitt ==
  In1 : Inport
  Constant2 : Constant
  Constant3 : Constant  Value=0
  Switch : Switch  Threshold=trgo_th_generator  SaturateOnIntegerOverflow=off  InputSameDT=off
  Out1 : Outport
  wires:
  Switch/1 -> Out1/1
  In1/1 -> Switch/2
  Constant3/1 -> Switch/1
  Constant2/1 -> Switch/3

== system two_time_domains/global timing/trgo-inv2/schmitt ==
  In1 : Inport
  Constant2 : Constant
  Constant3 : Constant  Value=0
  Switch : Switch  Threshold=trgo_th_generator  SaturateOnIntegerOverflow=off  InputSameDT=off
  Out1 : Outport
  wires:
  Constant2/1 -> Switch/3
  Constant3/1 -> Switch/1
  In1/1 -> Switch/2
  Switch/1 -> Out1/1

== system two_time_domains/pwm_alignment_ctrl/phase_compensation_1/alignment_eval_afe1 ==
  local_time : Inport
  master_time : Inport  Port=2
  Constant : Constant  Value=0
  Gain : Gain  Gain=-1
  Sum : Sum  Inputs=|+-
  pi : Subsystem  mask{kp=kp_align, ki=ki_align, lim_up=lim_up_align, lim_down=lim_down_align}
      mask prompts: ki "ki*ts"
      mask Display:
      | disp('pi()');
      | port_label('input', 1, 'u_ref');
      | port_label('input', 2, 'u');
      | port_label('output', 1, 'y');
  dp : Outport
  wires:
  master_time/1 -> Sum/1
  Sum/1 -> Gain/1
  Constant/1 -> pi/1(u_ref)
  local_time/1 -> Sum/2
  Gain/1 -> pi/2(u)
  pi/1(y) -> dp/1

== system two_time_domains/pwm_alignment_ctrl/phase_compensation_2/alignment_eval_afe1 ==
  local_time : Inport
  master_time : Inport  Port=2
  Constant : Constant  Value=0
  Gain : Gain  Gain=-1
  Sum : Sum  Inputs=|+-
  pi : Subsystem  mask{kp=kp_align, ki=ki_align, lim_up=lim_up_align, lim_down=lim_down_align}
      mask prompts: ki "ki*ts"
      mask Display:
      | disp('pi()');
      | port_label('input', 1, 'u_ref');
      | port_label('input', 2, 'u');
      | port_label('output', 1, 'y');
  dp : Outport
  wires:
  pi/1(y) -> dp/1
  master_time/1 -> Sum/1
  local_time/1 -> Sum/2
  Sum/1 -> Gain/1
  Constant/1 -> pi/1(u_ref)
  Gain/1 -> pi/2(u)

== system two_time_domains/pwm_alignment_ctrl/phase_compensation_3/alignment_eval_afe1 ==
  local_time : Inport
  master_time : Inport  Port=2
  Constant : Constant  Value=0
  Gain : Gain  Gain=-1
  Sum : Sum  Inputs=|+-
  pi : Subsystem  mask{kp=kp_align, ki=ki_align, lim_up=lim_up_align, lim_down=lim_down_align}
      mask prompts: ki "ki*ts"
      mask Display:
      | disp('pi()');
      | port_label('input', 1, 'u_ref');
      | port_label('input', 2, 'u');
      | port_label('output', 1, 'y');
  dp : Outport
  wires:
  master_time/1 -> Sum/1
  Sum/1 -> Gain/1
  Constant/1 -> pi/1(u_ref)
  local_time/1 -> Sum/2
  Gain/1 -> pi/2(u)
  pi/1(y) -> dp/1

== system two_time_domains/pwm_alignment_ctrl/phase_compensation_4/alignment_eval_afe1 ==
  local_time : Inport
  master_time : Inport  Port=2
  Constant : Constant  Value=0
  Gain : Gain  Gain=-1
  Sum : Sum  Inputs=|+-
  pi : Subsystem  mask{kp=kp_align, ki=ki_align, lim_up=lim_up_align, lim_down=lim_down_align}
      mask prompts: ki "ki*ts"
      mask Display:
      | disp('pi()');
      | port_label('input', 1, 'u_ref');
      | port_label('input', 2, 'u');
      | port_label('output', 1, 'y');
  dp : Outport
  wires:
  master_time/1 -> Sum/1
  Sum/1 -> Gain/1
  Constant/1 -> pi/1(u_ref)
  local_time/1 -> Sum/2
  Gain/1 -> pi/2(u)
  pi/1(y) -> dp/1

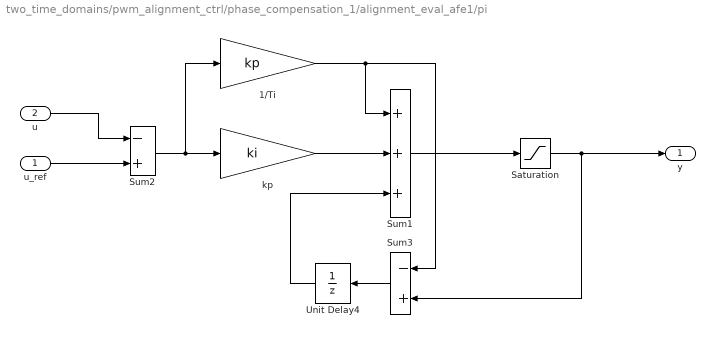
== system two_time_domains/pwm_alignment_ctrl/phase_compensation_1/alignment_eval_afe1/pi ==
  u_ref : Inport
  u : Inport  Port=2
  1/Ti : Gain  Gain=kp  SaturateOnIntegerOverflow=on  OutDataTypeStr=Inherit: Same as input  ParamDataTypeStr=Inherit: Same as input
  Saturation : Saturate  UpperLimit=lim_up  LowerLimit=lim_down
  Sum1 : Sum  Inputs=+++  SaturateOnIntegerOverflow=on
  Sum2 : Sum  Inputs=-+  SaturateOnIntegerOverflow=on
  Sum3 : Sum  Inputs=-+  SaturateOnIntegerOverflow=on
  Unit Delay4 : UnitDelay  SampleTime=-1  HasFrameUpgradeWarning=on
  kp : Gain  Gain=ki  SaturateOnIntegerOverflow=on  OutDataTypeStr=Inherit: Same as input  ParamDataTypeStr=Inherit: Same as input
  y : Outport
  wires:
  1/Ti/1 -> Sum1/1, Sum3/1
  kp/1 -> Sum1/2
  Sum3/1 -> Unit Delay4/1
  Unit Delay4/1 -> Sum1/3
  u_ref/1 -> Sum2/2
  u/1 -> Sum2/1
  Sum2/1 -> kp/1, 1/Ti/1
  Sum1/1 -> Saturation/1
  Saturation/1 -> Sum3/2, y/1

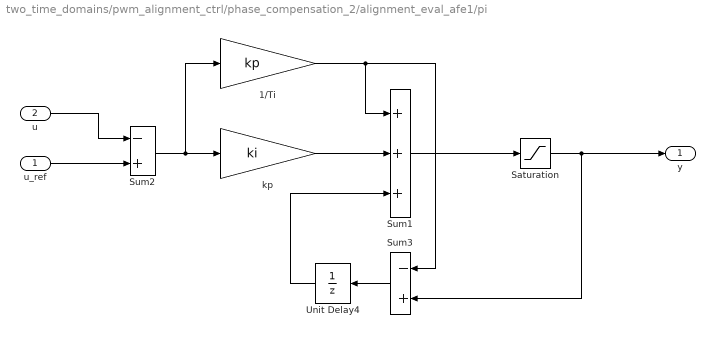
== system two_time_domains/pwm_alignment_ctrl/phase_compensation_2/alignment_eval_afe1/pi ==
  u_ref : Inport
  u : Inport  Port=2
  1/Ti : Gain  Gain=kp  SaturateOnIntegerOverflow=on  OutDataTypeStr=Inherit: Same as input  ParamDataTypeStr=Inherit: Same as input
  Saturation : Saturate  UpperLimit=lim_up  LowerLimit=lim_down
  Sum1 : Sum  Inputs=+++  SaturateOnIntegerOverflow=on
  Sum2 : Sum  Inputs=-+  SaturateOnIntegerOverflow=on
  Sum3 : Sum  Inputs=-+  SaturateOnIntegerOverflow=on
  Unit Delay4 : UnitDelay  SampleTime=-1  HasFrameUpgradeWarning=on
  kp : Gain  Gain=ki  SaturateOnIntegerOverflow=on  OutDataTypeStr=Inherit: Same as input  ParamDataTypeStr=Inherit: Same as input
  y : Outport
  wires:
  1/Ti/1 -> Sum1/1, Sum3/1
  kp/1 -> Sum1/2
  Sum3/1 -> Unit Delay4/1
  Unit Delay4/1 -> Sum1/3
  u_ref/1 -> Sum2/2
  u/1 -> Sum2/1
  Sum2/1 -> kp/1, 1/Ti/1
  Sum1/1 -> Saturation/1
  Saturation/1 -> Sum3/2, y/1

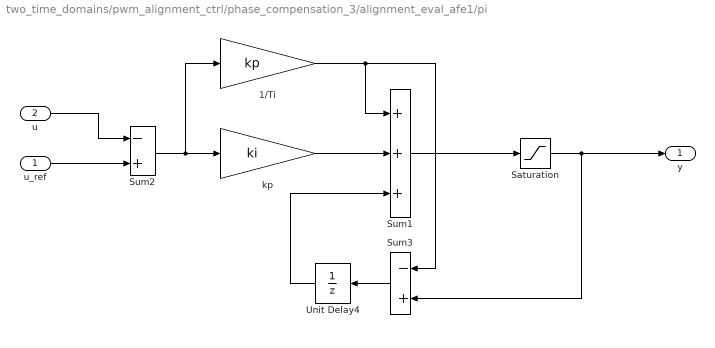
== system two_time_domains/pwm_alignment_ctrl/phase_compensation_3/alignment_eval_afe1/pi ==
  u_ref : Inport
  u : Inport  Port=2
  1/Ti : Gain  Gain=kp  SaturateOnIntegerOverflow=on  OutDataTypeStr=Inherit: Same as input  ParamDataTypeStr=Inherit: Same as input
  Saturation : Saturate  UpperLimit=lim_up  LowerLimit=lim_down
  Sum1 : Sum  Inputs=+++  SaturateOnIntegerOverflow=on
  Sum2 : Sum  Inputs=-+  SaturateOnIntegerOverflow=on
  Sum3 : Sum  Inputs=-+  SaturateOnIntegerOverflow=on
  Unit Delay4 : UnitDelay  SampleTime=-1  HasFrameUpgradeWarning=on
  kp : Gain  Gain=ki  SaturateOnIntegerOverflow=on  OutDataTypeStr=Inherit: Same as input  ParamDataTypeStr=Inherit: Same as input
  y : Outport
  wires:
  1/Ti/1 -> Sum1/1, Sum3/1
  kp/1 -> Sum1/2
  Sum3/1 -> Unit Delay4/1
  Unit Delay4/1 -> Sum1/3
  u_ref/1 -> Sum2/2
  u/1 -> Sum2/1
  Sum2/1 -> kp/1, 1/Ti/1
  Sum1/1 -> Saturation/1
  Saturation/1 -> Sum3/2, y/1

== system two_time_domains/pwm_alignment_ctrl/phase_compensation_4/alignment_eval_afe1/pi ==
  u_ref : Inport
  u : Inport  Port=2
  1/Ti : Gain  Gain=kp  SaturateOnIntegerOverflow=on  OutDataTypeStr=Inherit: Same as input  ParamDataTypeStr=Inherit: Same as input
  Saturation : Saturate  UpperLimit=lim_up  LowerLimit=lim_down
  Sum1 : Sum  Inputs=+++  SaturateOnIntegerOverflow=on
  Sum2 : Sum  Inputs=-+  SaturateOnIntegerOverflow=on
  Sum3 : Sum  Inputs=-+  SaturateOnIntegerOverflow=on
  Unit Delay4 : UnitDelay  SampleTime=-1  HasFrameUpgradeWarning=on
  kp : Gain  Gain=ki  SaturateOnIntegerOverflow=on  OutDataTypeStr=Inherit: Same as input  ParamDataTypeStr=Inherit: Same as input
  y : Outport
  wires:
  1/Ti/1 -> Sum1/1, Sum3/1
  kp/1 -> Sum1/2
  Sum3/1 -> Unit Delay4/1
  Unit Delay4/1 -> Sum1/3
  u_ref/1 -> Sum2/2
  u/1 -> Sum2/1
  Sum2/1 -> kp/1, 1/Ti/1
  Sum1/1 -> Saturation/1
  Saturation/1 -> Sum3/2, y/1

== matlab function two_time_domains/pwm domains/PWM generator INV 1/MATLAB Function ==
  data: t input; y output; phase input; period input
function y = trgo(t,phase,period)
x = sin(2*pi/period*t - phase -pi/2);
y = asin(x);

== matlab function two_time_domains/pwm domains/PWM generator INV 2/MATLAB Function ==
  data: t input; y output; phase input; period input
function y = trgo(t,phase,period)
x = sin(2*pi/period*t - phase -pi/2);
y = asin(x);

== matlab function two_time_domains/pwm domains/PWM generator AFE 1/MATLAB Function ==
  data: t input; y output; phase input; period input
function y = trgo(t,phase,period)
x = sin(2*pi/period*t - phase -pi/2);
y = asin(x);

== matlab function two_time_domains/pwm domains/PWM generator AFE 2/MATLAB Function ==
  data: t input; y output; phase input; period input
function y = trgo(t,phase,period)
x = sin(2*pi/period*t - phase -pi/2);
y = asin(x);
